simulink model "PV_Boost_Converter_PWM"  (R2020a)
settings: Solver=FixedStepAuto  StartTime=0.0  StopTime=0.5  FixedStep=1e-6  RelTol=1e-3
values from neighbouring files (symbols this model uses):
  Eg = 1.1    [data.m]
  Isc = 8.21    [data.m]
  k = 1.38*((10)^-23)    (= 1.38e-23)    [data.m]
  ki = 0.0032    [data.m]
  n = 1.3    [data.m]
  Ns = 54    [data.m]
  q = 1.6*((10)^-19)    (= 1.6e-19)    [data.m]
  Rs = 0.221    [data.m]
  Rsh = 415.405    [data.m]
  Tn = 298    [data.m]
  Voc = 32.9    [data.m]
libraries: powerlib x27, fuzblock x2, powerlib_meascontrol x2, re_lib x1
settings Model: Creator=Khojasteh Mirza  LastModifiedBy=Khojasteh Mirza

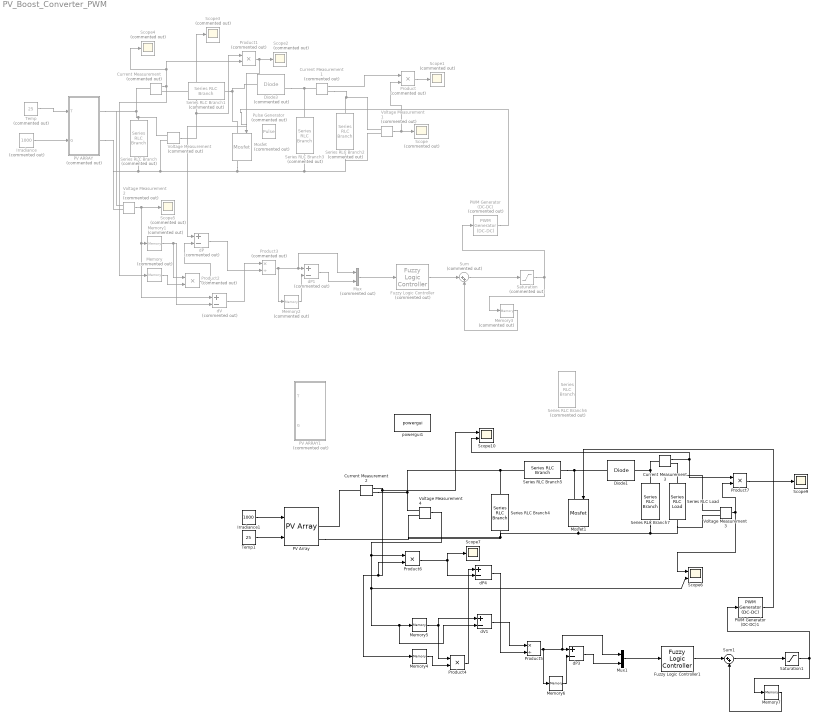
== system PV_Boost_Converter_PWM ==
  Current Measurement : powerlib/Measurements/Current Measurement  Commented=on  PhasorSimulation=off  OutputType=Complex  PSBequivalent=0
  Current Measurement1 : powerlib/Measurements/Current Measurement  Commented=on  PhasorSimulation=off  OutputType=Complex  PSBequivalent=0
  Current Measurement2 : powerlib/Measurements/Current Measurement  PhasorSimulation=off  OutputType=Complex  PSBequivalent=0
  Current Measurement3 : powerlib/Measurements/Current Measurement  PhasorSimulation=off  OutputType=Complex  PSBequivalent=0
  Diode1 : powerlib/Power Electronics/Diode  Ron=0.001  Lon=0  Vf=0.8  IC=0  UseSnubber=0  Rs=500  Cs=250e-9  Measurements=off
  Diode3 : powerlib/Power Electronics/Diode  Commented=on  Ron=0.001  Lon=0  Vf=0.8  IC=0  UseSnubber=0  Rs=500  Cs=250e-9  Measurements=on
  Fuzzy Logic Controller : fuzblock/Fuzzy Logic  Controller  Commented=on  FIS='fuzzy_mppt.fis'  OutputSampleNumber=101  DataType=double  FuzzifiedInputs=off  RuleFiringStrengths=off  RuleOutputs=off  AggregatedOutputs=off  SimulateUsing=Interpreted execution  OutOfRangeInputValueMessage=warning  NoRuleFiredMessage=warning  EmptyOutputFuzzySetMessage=warning
  Fuzzy Logic Controller1 : fuzblock/Fuzzy Logic  Controller  FIS='fuzzy_mppt.fis'  OutputSampleNumber=101  DataType=double  FuzzifiedInputs=off  RuleFiringStrengths=off  RuleOutputs=off  AggregatedOutputs=off  SimulateUsing=Interpreted execution  OutOfRangeInputValueMessage=warning  NoRuleFiredMessage=warning  EmptyOutputFuzzySetMessage=warning
  Irradiance : Constant  Commented=on  Value=1000
  Irradiance1 : Constant  Value=1000
  Memory{,1..3} (4 alike) : Memory  Commented=on
  Memory{4..7} (4 alike) : Memory
  Mosfet : powerlib/Power Electronics/Mosfet  Commented=on  Ron=0.1  Lon=0  Rd=0.01  Vfd=0  IC=0  Rs=1e5  Cs=inf  Measurements=on
  Mosfet1 : powerlib/Power Electronics/Mosfet  Ron=0.1  Lon=0  Rd=0.01  Vfd=0  IC=0  Rs=1e5  Cs=inf  Measurements=off
  Mux : Mux  Commented=on  Inputs=2
  Mux1 : Mux  Inputs=2
  PV ARRAY : Subsystem  Commented=on
  PV ARRAY1 : Subsystem  Commented=on
  PV Array : re_lib/Solar/PV Array  Npar=1  Nser=1  PlotType=array @ 25 deg.C & specified irradiances  S_vec=[1000]  Temp_C_vec=[800]  ModuleName=Kyocera Solar KC200GT  PlotWhenSelected=off  Pm=200.143  Ncell=54  Voc=32.9  Isc=8.21  Vm=26.3  Im=7.61  beta_Voc_pc=-0.35502  alpha_Isc_pc=0.06  beta_Voc=-0.1168  alpha_Isc=0.004926  IL=8.2288  I0=2.3246e-10  nI=0.97736  Rsh=150.6921  Rs=0.34483  RobustModel=off  RobustCellTemperature=25  BAL=on  Tc=1e-6  Tfilter=5e-5
  PWM Generator (DC-DC) : powerlib_meascontrol/Pulse & Signal Generators/PWM Generator (DC-DC)  Commented=on  Fsw=5000  Ts=0
  PWM Generator (DC-DC)1 : powerlib_meascontrol/Pulse & Signal Generators/PWM Generator (DC-DC)  Fsw=5000  Ts=0
  Product : Product  Commented=on
  Product1 : Product  Commented=on
  Product2 : Product  Commented=on
  Product3 : Product  Commented=on  Inputs=*/
  Product4 : Product
  Product5 : Product  Inputs=*/
  Product6 : Product
  Product7 : Product
  Pulse Generator : DiscretePulseGenerator  Commented=on  PulseType=Time based  Period=0.00004  PulseWidth=10
  Saturation : Saturate  Commented=on
  Saturation1 : Saturate
  Scope{,1..5} (6 alike) : Scope  Commented=on
  Scope10 : Scope  NumInputPorts=2
  Scope6 : Scope  NumInputPorts=2
  Scope7 : Scope
  Scope9 : Scope
  Series RLC Branch : powerlib/Elements/Series RLC Branch  Commented=on  LConnTagsString=__new0  RConnTagsString=__new0  BranchType=C  Resistance=1  Inductance=1e-3  SetiL0=off  InitialCurrent=0  Capacitance=1e-6  Setx0=off  InitialVoltage=0  Measurements=None
  Series RLC Branch1 : powerlib/Elements/Series RLC Branch  Commented=on  LConnTagsString=__new0  RConnTagsString=__new0  BranchType=L  Resistance=1  Inductance=650e-6  SetiL0=off  InitialCurrent=0  Capacitance=1e-6  Setx0=off  InitialVoltage=0  Measurements=None
  Series RLC Branch2 : powerlib/Elements/Series RLC Branch  Commented=on  LConnTagsString=__new0  RConnTagsString=__new0  BranchType=R  Resistance=10  Inductance=1e-3  SetiL0=off  InitialCurrent=0  Capacitance=1e-6  Setx0=off  InitialVoltage=0  Measurements=None
  Series RLC Branch3 : powerlib/Elements/Series RLC Branch  Commented=on  LConnTagsString=__new0  RConnTagsString=__new0  BranchType=C  Resistance=1  Inductance=1e-3  SetiL0=off  InitialCurrent=0  Capacitance=30e-6  Setx0=off  InitialVoltage=0  Measurements=None
  Series RLC Branch4 : powerlib/Elements/Series RLC Branch  LConnTagsString=__new0  RConnTagsString=__new0  BranchType=C  Resistance=1  Inductance=1e-3  SetiL0=off  InitialCurrent=0  Capacitance=4000e-6  Setx0=off  InitialVoltage=0  Measurements=None
  Series RLC Branch5 : powerlib/Elements/Series RLC Branch  LConnTagsString=__new0  RConnTagsString=__new0  BranchType=L  Resistance=1  Inductance=1e-4  SetiL0=off  InitialCurrent=0  Capacitance=1e-6  Setx0=off  InitialVoltage=0  Measurements=None
  Series RLC Branch6 : powerlib/Elements/Series RLC Branch  Commented=on  LConnTagsString=__new0  RConnTagsString=__new0  BranchType=R  Resistance=10  Inductance=1e-3  SetiL0=off  InitialCurrent=0  Capacitance=1e-6  Setx0=off  InitialVoltage=0  Measurements=None
  Series RLC Branch7 : powerlib/Elements/Series RLC Branch  LConnTagsString=__new0  RConnTagsString=__new0  BranchType=C  Resistance=1  Inductance=1e-3  SetiL0=off  InitialCurrent=0  Capacitance=50e-6  Setx0=off  InitialVoltage=0  Measurements=None
  Series RLC Load : powerlib/Elements/Series RLC Load  LConnTagsString=a  RConnTagsString=__new0  NominalVoltage=30  NominalFrequency=50  ActivePower=120  InductivePower=0  CapacitivePower=0  Setx0=off  InitialVoltage=0  SetiL0=off  InitialCurrent=0  Measurements=None  LoadType=constant Z
  Sum : Sum  Commented=on  Inputs=|++
  Sum1 : Sum  Inputs=|++
  Temp : Constant  Commented=on  Value=25
  Temp1 : Constant  Value=25
  Voltage Measurement : powerlib/Measurements/Voltage Measurement  Commented=on  PhasorSimulation=off  OutputType=Complex  PSBequivalent=0
  Voltage Measurement1 : powerlib/Measurements/Voltage Measurement  Commented=on  PhasorSimulation=off  OutputType=Complex  PSBequivalent=0
  Voltage Measurement2 : powerlib/Measurements/Voltage Measurement  Commented=on  PhasorSimulation=off  OutputType=Complex  PSBequivalent=0
  Voltage Measurement3 : powerlib/Measurements/Voltage Measurement  PhasorSimulation=off  OutputType=Complex  PSBequivalent=0
  Voltage Measurement4 : powerlib/Measurements/Voltage Measurement  PhasorSimulation=off  OutputType=Complex  PSBequivalent=0
  dP : Sum  Commented=on  Inputs=+-
  dP1 : Sum  Commented=on  Inputs=+-
  dP3 : Sum  Inputs=+-
  dP4 : Sum  Inputs=+-
  dV : Sum  Commented=on  Inputs=+-
  dV1 : Sum  Inputs=+-
  powergui1 : powerlib/powergui  Priority=1  SimulationMode=Discrete  SampleTime=5e-5  frequency=60  Iterations=50  frequencyindice=0  Pbase=100e6  ErrMax=1e-4  UnitsV=kV  UnitsW=MW  buscounter=0  FunctionMessages=off  echomessages=off  EnableUseOfTLC=off  CurrentSourceSwitches=off  DisableSnubberDevices=off  DisableRonSwitches=off  DisableVfSwitches=off  DisplayEquations=off  AutomaticDiscreteSolvers=off  SolverType=Tustin/Backward Euler (TBE)  Interpol=off  ExternalGateDelay=off  methode=off  Ts=100  x0status=blocks  SPID=on  SwTol=0  HookPort=off  NonlinearTolerance=1e-4  nMaxIteration=100  ContinueOnMaxIteration=off  RestoreLinks=warning  ResistiveCurrentMeasurement=off  Frange=[0:2:500]  Ylog=off  Xlog=on  ShowGrid=off  save=off  variable=ZData  structure=0  ZoomFFT=off  StartTime=0.0  cycles=1  DisplayStyle=1  fundamental=60  FreqAxis=off  MaxFrequency=1000  frequencyindicesteady=1  RmsSteady=1  display=off
  wires:
  Temp/1 -> PV ARRAY/1(T)
  Irradiance/1 -> PV ARRAY/2(G)
  Voltage Measurement1/1 -> Product/2, Scope/1
  Current Measurement1/1 -> Product/1
  Product/1 -> Scope1/1
  Product1/1 -> dP/1, Scope2/1
  Voltage Measurement/1 -> Scope3/1, Product1/1
  Current Measurement/1 -> Scope4/1, Product1/2, Memory/1
  Voltage Measurement2/1 -> dV/1, Memory1/1, Scope5/1
  Memory1/1 -> dV/2, Product2/1
  Memory/1 -> Product2/2
  Product2/1 -> dP/2
  dV/1 -> Product3/1
  dP/1 -> Product3/2
  Product3/1 -> Memory2/1, Mux/1, dP1/1
  Memory2/1 -> dP1/2
  dP1/1 -> Mux/2
  Mux/1 -> Fuzzy Logic Controller/1
  Fuzzy Logic Controller/1 -> Sum/1
  Sum/1 -> Saturation/1
  Saturation/1 -> PWM Generator (DC-DC)/1, Memory3/1
  Memory3/1 -> Sum/2
  PWM Generator (DC-DC)/1 -> Mosfet/1
  Memory4/1 -> Product4/2
  Memory7/1 -> Sum1/2
  Sum1/1 -> Saturation1/1
  Product4/1 -> dP4/1
  dP3/1 -> Mux1/2
  Saturation1/1 -> PWM Generator (DC-DC)1/1, Memory7/1
  dV1/1 -> Product5/1
  Memory6/1 -> dP3/2
  Mux1/1 -> Fuzzy Logic Controller1/1
  Fuzzy Logic Controller1/1 -> Sum1/1
  Memory5/1 -> dV1/1, Product4/1
  Product5/1 -> Memory6/1, Mux1/1, dP3/1
  Current Measurement2/1 -> Scope10/1, Memory4/1, Product6/2
  Product6/1 -> Scope7/1, dP4/2
  dP4/1 -> Product5/2
  PWM Generator (DC-DC)1/1 -> Mosfet1/1
  Voltage Measurement3/1 -> Product7/2, Scope6/1
  Irradiance1/1 -> PV Array/1
  Temp1/1 -> PV Array/2
  Current Measurement3/1 -> Product7/1, Scope10/2
  Product7/1 -> Scope9/1
  Voltage Measurement4/1 -> Scope6/2, dV1/2, Memory5/1, Product6/1
  connections:
  Current Measurement/LConn1 -- Voltage Measurement2/LConn1 -- PV ARRAY/RConn1 -- Series RLC Branch/LConn1 -- Voltage Measurement/LConn1
  Series RLC Branch1/LConn1 -- Current Measurement/RConn1
  Series RLC Branch2/LConn1 -- Current Measurement1/RConn1 -- Voltage Measurement1/LConn1
  Series RLC Branch3/LConn1 -- Diode3/RConn1 -- Current Measurement1/LConn1
  Series RLC Branch3/RConn1 -- Mosfet/RConn1 -- Series RLC Branch/RConn1 -- PV ARRAY/RConn2 -- Voltage Measurement2/LConn2 -- Voltage Measurement/LConn2 -- Voltage Measurement1/LConn2 -- Series RLC Branch2/RConn1
  Series RLC Branch1/RConn1 -- Diode3/LConn1 -- Mosfet/LConn1
  Series RLC Branch5/RConn1 -- Diode1/LConn1 -- Mosfet1/LConn1
  Voltage Measurement3/LConn1 -- Current Measurement3/RConn1 -- Series RLC Load/LConn1
  Current Measurement2/RConn1 -- Series RLC Branch4/LConn1 -- Series RLC Branch5/LConn1 -- Voltage Measurement4/LConn1
  Series RLC Branch4/RConn1 -- Voltage Measurement4/LConn2 -- PV Array/RConn2 -- Voltage Measurement3/LConn2 -- Series RLC Load/RConn1 -- Series RLC Branch7/RConn1 -- Mosfet1/RConn1
  Current Measurement2/LConn1 -- PV Array/RConn1
  Series RLC Branch7/LConn1 -- Current Measurement3/LConn1 -- Diode1/RConn1

== system PV_Boost_Converter_PWM/PV ARRAY ==
  T : Inport
  G : Inport  Port=2
  Controlled Current Source : powerlib/Electrical Sources/Controlled Current Source  Initialize=on  Source_Type=AC  Amplitude=0  Phase=0  Frequency=0  Measurements=None
  PV Module : Subsystem
  Voltage Measurement : powerlib/Measurements/Voltage Measurement  PhasorSimulation=off  OutputType=Complex  PSBequivalent=0
  + : PMIOPort  Side=Right
  - : PMIOPort  Port=2  Side=Right
  wires:
  G/1 -> PV Module/2(G)
  Voltage Measurement/1 -> PV Module/3(Varray)
  T/1 -> PV Module/1(T)
  PV Module/1(I) -> Controlled Current Source/1
  connections:
  Controlled Current Source/LConn1 -- -/RConn1 -- Voltage Measurement/LConn2
  Controlled Current Source/RConn1 -- +/RConn1 -- Voltage Measurement/LConn1

== system PV_Boost_Converter_PWM/PV ARRAY1 ==
  T : Inport
  G : Inport  Port=2
  Controlled Current Source : powerlib/Electrical Sources/Controlled Current Source  Initialize=on  Source_Type=AC  Amplitude=0  Phase=0  Frequency=0  Measurements=None
  PV Module : Subsystem
  Voltage Measurement : powerlib/Measurements/Voltage Measurement  PhasorSimulation=off  OutputType=Complex  PSBequivalent=0
  + : PMIOPort  Side=Right
  - : PMIOPort  Port=2  Side=Right
  wires:
  G/1 -> PV Module/2(G)
  Voltage Measurement/1 -> PV Module/3(Varray)
  T/1 -> PV Module/1(T)
  PV Module/1(I) -> Controlled Current Source/1
  connections:
  Controlled Current Source/LConn1 -- -/RConn1 -- Voltage Measurement/LConn2
  Controlled Current Source/RConn1 -- +/RConn1 -- Voltage Measurement/LConn1

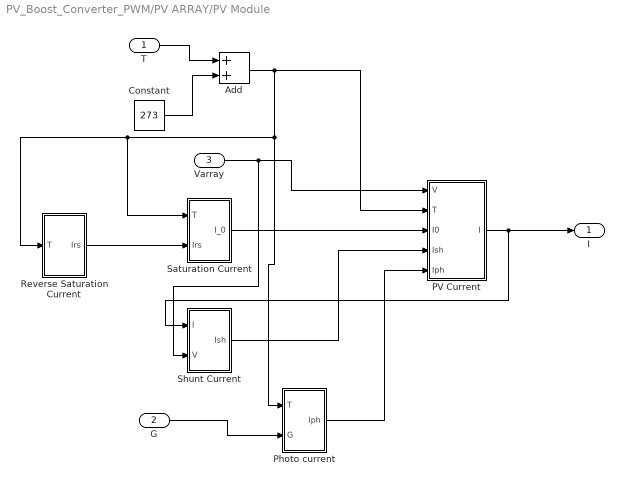
== system PV_Boost_Converter_PWM/PV ARRAY/PV Module ==
  T : Inport
  G : Inport  Port=2
  Varray : Inport  Port=3
  Add : Sum
  Constant : Constant  Value=273
  PV Current : Subsystem
  Photo current : Subsystem
  Reverse Saturation Current : Subsystem
  Saturation Current : Subsystem
  Shunt Current : Subsystem
  I : Outport
  wires:
  Shunt Current/1(Ish) -> PV Current/4(Ish)
  Varray/1 -> Shunt Current/2(V), PV Current/1(V)
  Reverse Saturation Current/1(Irs) -> Saturation Current/2(Irs)
  Saturation Current/1(I_0) -> PV Current/3(I0)
  Constant/1 -> Add/2
  G/1 -> Photo current/2(G)
  T/1 -> Add/1
  PV Current/1(I) -> I/1, Shunt Current/1(I)
  Photo current/1(Iph) -> PV Current/5(Iph)
  Add/1 -> Saturation Current/1(T), Reverse Saturation Current/1(T), Photo current/1(T), PV Current/2(T)

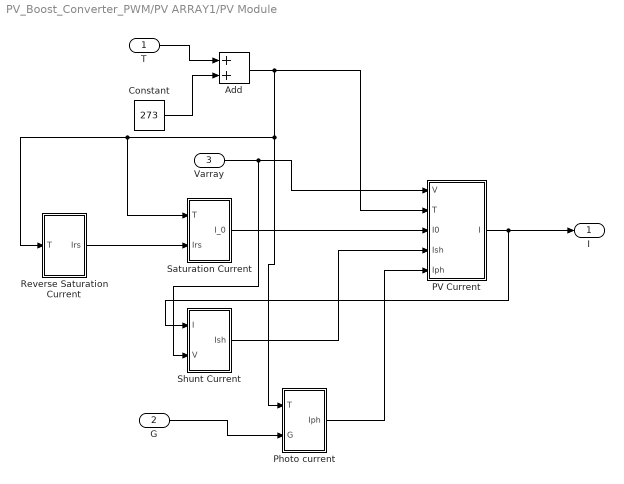
== system PV_Boost_Converter_PWM/PV ARRAY1/PV Module ==
  T : Inport
  G : Inport  Port=2
  Varray : Inport  Port=3
  Add : Sum
  Constant : Constant  Value=273
  PV Current : Subsystem
  Photo current : Subsystem
  Reverse Saturation Current : Subsystem
  Saturation Current : Subsystem
  Shunt Current : Subsystem
  I : Outport
  wires:
  Shunt Current/1(Ish) -> PV Current/4(Ish)
  Varray/1 -> Shunt Current/2(V), PV Current/1(V)
  Reverse Saturation Current/1(Irs) -> Saturation Current/2(Irs)
  Saturation Current/1(I_0) -> PV Current/3(I0)
  Constant/1 -> Add/2
  G/1 -> Photo current/2(G)
  T/1 -> Add/1
  PV Current/1(I) -> I/1, Shunt Current/1(I)
  Photo current/1(Iph) -> PV Current/5(Iph)
  Add/1 -> Saturation Current/1(T), Reverse Saturation Current/1(T), Photo current/1(T), PV Current/2(T)

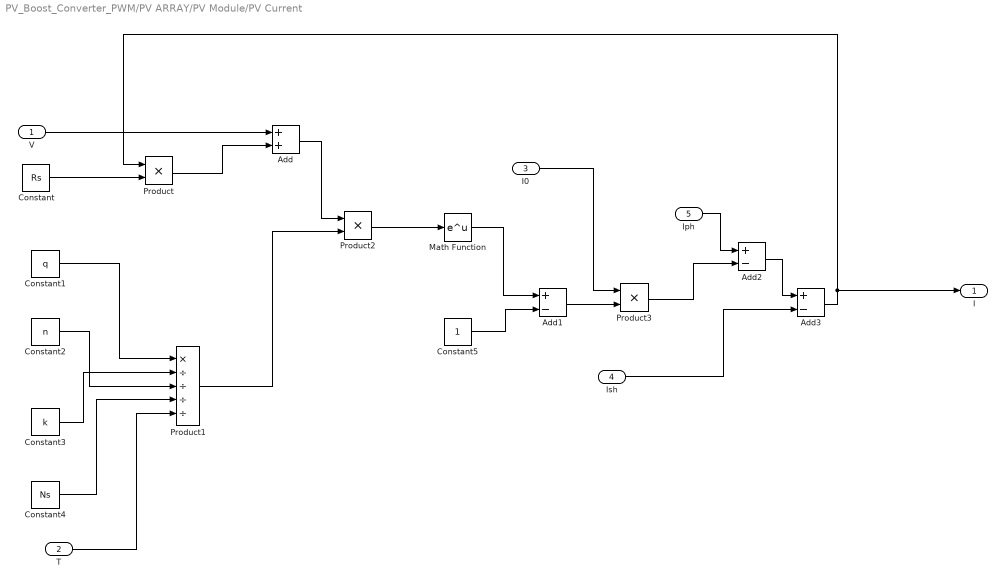
== system PV_Boost_Converter_PWM/PV ARRAY/PV Module/PV Current ==
  V : Inport
  T : Inport  Port=2
  I0 : Inport  Port=3
  Ish : Inport  Port=4
  Iph : Inport  Port=5
  Add : Sum
  Add1 : Sum  Inputs=+-
  Add2 : Sum  Inputs=+-
  Add3 : Sum  Inputs=+-
  Constant : Constant  Value=Rs
  Constant1 : Constant  Value=q
  Constant2 : Constant  Value=n
  Constant3 : Constant  Value=k
  Constant4 : Constant  Value=Ns
  Constant5 : Constant
  Math Function : Math  SaturateOnIntegerOverflow=on
  Product : Product
  Product1 : Product  Inputs=*////
  Product2 : Product
  Product3 : Product
  I : Outport
  wires:
  Constant3/1 -> Product1/2
  Constant/1 -> Product/2
  Math Function/1 -> Add1/1
  Iph/1 -> Add2/1
  Product2/1 -> Math Function/1
  I0/1 -> Product3/1
  Ish/1 -> Add3/2
  Product/1 -> Add/2
  Constant4/1 -> Product1/4
  Add/1 -> Product2/1
  Add3/1 -> I/1, Product/1
  Add1/1 -> Product3/2
  Constant2/1 -> Product1/3
  Add2/1 -> Add3/1
  T/1 -> Product1/5
  Product3/1 -> Add2/2
  V/1 -> Add/1
  Constant1/1 -> Product1/1
  Constant5/1 -> Add1/2
  Product1/1 -> Product2/2

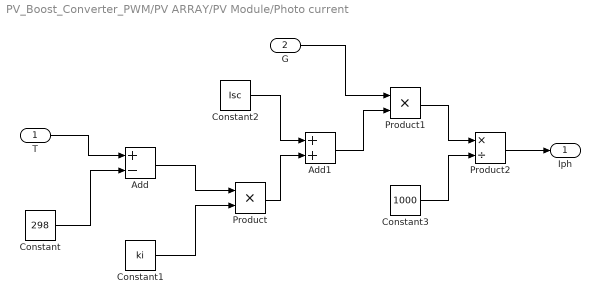
== system PV_Boost_Converter_PWM/PV ARRAY/PV Module/Photo current ==
  T : Inport
  G : Inport  Port=2
  Add : Sum  Inputs=+-
  Add1 : Sum
  Constant : Constant  Value=298
  Constant1 : Constant  Value=ki
  Constant2 : Constant  Value=Isc
  Constant3 : Constant  Value=1000
  Product : Product
  Product1 : Product
  Product2 : Product  Inputs=*/
  Iph : Outport
  wires:
  Add/1 -> Product/1
  T/1 -> Add/1
  Constant2/1 -> Add1/1
  Constant/1 -> Add/2
  Product/1 -> Add1/2
  Constant1/1 -> Product/2
  G/1 -> Product1/1
  Constant3/1 -> Product2/2
  Add1/1 -> Product1/2
  Product1/1 -> Product2/1
  Product2/1 -> Iph/1

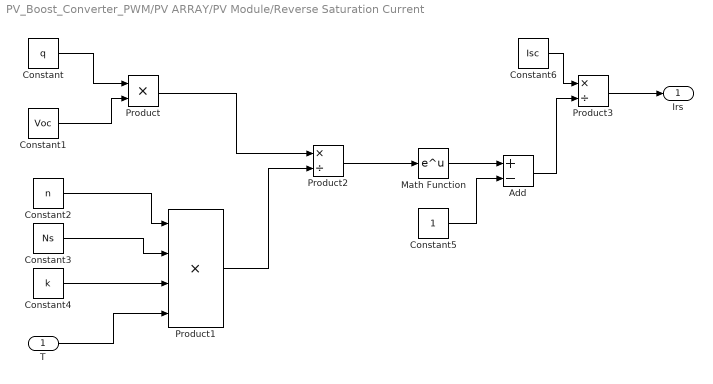
== system PV_Boost_Converter_PWM/PV ARRAY/PV Module/Reverse Saturation Current ==
  T : Inport
  Add : Sum  Inputs=+-
  Constant : Constant  Value=q
  Constant1 : Constant  Value=Voc
  Constant2 : Constant  Value=n
  Constant3 : Constant  Value=Ns
  Constant4 : Constant  Value=k
  Constant5 : Constant
  Constant6 : Constant  Value=Isc
  Math Function : Math  SaturateOnIntegerOverflow=on
  Product : Product
  Product1 : Product  Inputs=4
  Product2 : Product  Inputs=*/
  Product3 : Product  Inputs=*/
  Irs : Outport
  wires:
  Constant6/1 -> Product3/1
  Add/1 -> Product3/2
  Constant5/1 -> Add/2
  Constant3/1 -> Product1/2
  Product3/1 -> Irs/1
  Product1/1 -> Product2/2
  Math Function/1 -> Add/1
  Product/1 -> Product2/1
  Constant2/1 -> Product1/1
  Product2/1 -> Math Function/1
  Constant/1 -> Product/1
  Constant1/1 -> Product/2
  T/1 -> Product1/4
  Constant4/1 -> Product1/3

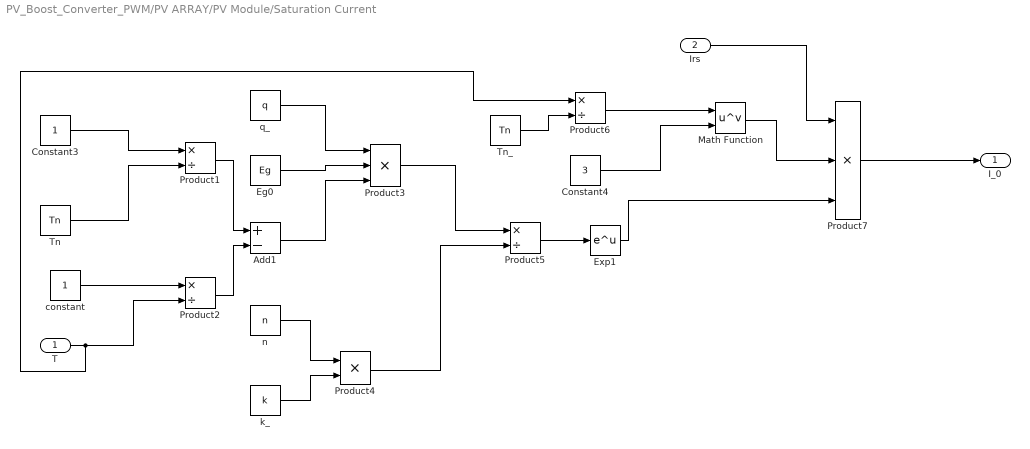
== system PV_Boost_Converter_PWM/PV ARRAY/PV Module/Saturation Current ==
  T : Inport
  Irs : Inport  Port=2
  Add1 : Sum  Inputs=+-
  Constant3 : Constant
  Constant4 : Constant  Value=3
  Eg0 : Constant  Value=Eg
  Exp1 : Math  SaturateOnIntegerOverflow=on
  Math Function : Math  Operator=pow  SaturateOnIntegerOverflow=on
  Product{1..2,5..6} (4 alike) : Product  Inputs=*/
  Product3 : Product  Inputs=***
  Product4 : Product  Inputs=**
  Product7 : Product  Inputs=3
  Tn : Constant  Value=Tn
  Tn_ : Constant  Value=Tn
  constant : Constant
  k_ : Constant  Value=k
  n : Constant  Value=n
  q_ : Constant  Value=q
  I_0 : Outport
  wires:
  T/1 -> Product2/2, Product6/1
  Product1/1 -> Add1/1
  constant/1 -> Product2/1
  Irs/1 -> Product7/1
  Tn_/1 -> Product6/2
  Product5/1 -> Exp1/1
  Product3/1 -> Product5/1
  q_/1 -> Product3/1
  Exp1/1 -> Product7/3
  Product2/1 -> Add1/2
  Product4/1 -> Product5/2
  Constant4/1 -> Math Function/2
  Math Function/1 -> Product7/2
  Tn/1 -> Product1/2
  Product6/1 -> Math Function/1
  k_/1 -> Product4/2
  Constant3/1 -> Product1/1
  Eg0/1 -> Product3/2
  n/1 -> Product4/1
  Add1/1 -> Product3/3
  Product7/1 -> I_0/1

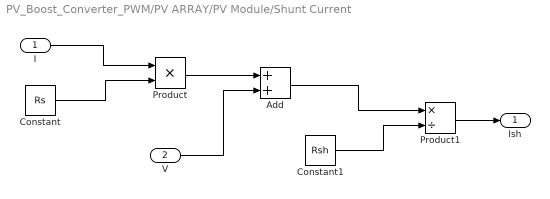
== system PV_Boost_Converter_PWM/PV ARRAY/PV Module/Shunt Current ==
  I : Inport
  V : Inport  Port=2
  Add : Sum
  Constant : Constant  Value=Rs
  Constant1 : Constant  Value=Rsh
  Product : Product
  Product1 : Product  Inputs=*/
  Ish : Outport
  wires:
  Product1/1 -> Ish/1
  Constant/1 -> Product/2
  Constant1/1 -> Product1/2
  V/1 -> Add/2
  Product/1 -> Add/1
  Add/1 -> Product1/1
  I/1 -> Product/1

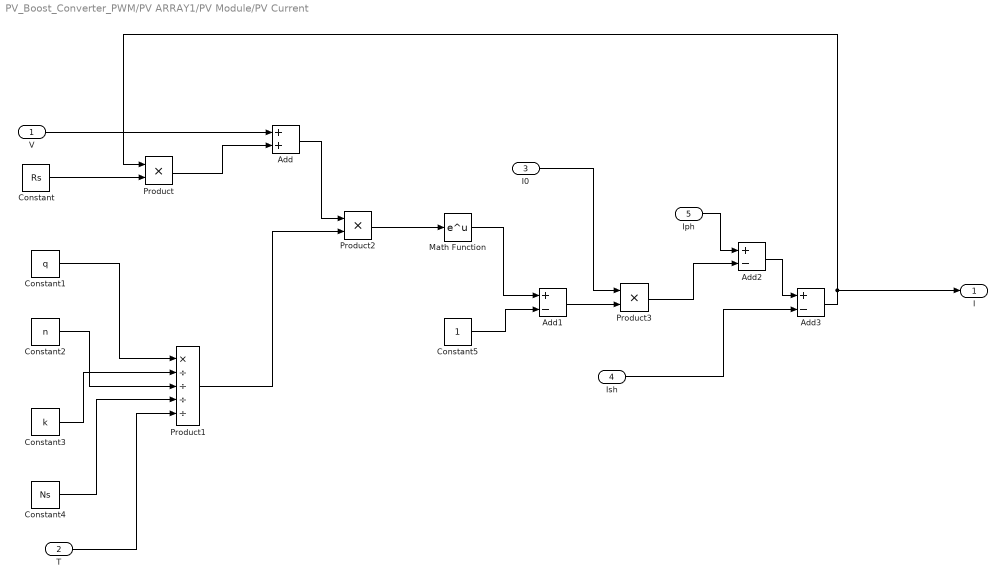
== system PV_Boost_Converter_PWM/PV ARRAY1/PV Module/PV Current ==
  V : Inport
  T : Inport  Port=2
  I0 : Inport  Port=3
  Ish : Inport  Port=4
  Iph : Inport  Port=5
  Add : Sum
  Add1 : Sum  Inputs=+-
  Add2 : Sum  Inputs=+-
  Add3 : Sum  Inputs=+-
  Constant : Constant  Value=Rs
  Constant1 : Constant  Value=q
  Constant2 : Constant  Value=n
  Constant3 : Constant  Value=k
  Constant4 : Constant  Value=Ns
  Constant5 : Constant
  Math Function : Math  SaturateOnIntegerOverflow=on
  Product : Product
  Product1 : Product  Inputs=*////
  Product2 : Product
  Product3 : Product
  I : Outport
  wires:
  Constant3/1 -> Product1/2
  Constant/1 -> Product/2
  Math Function/1 -> Add1/1
  Iph/1 -> Add2/1
  Product2/1 -> Math Function/1
  I0/1 -> Product3/1
  Ish/1 -> Add3/2
  Product/1 -> Add/2
  Constant4/1 -> Product1/4
  Add/1 -> Product2/1
  Add3/1 -> I/1, Product/1
  Add1/1 -> Product3/2
  Constant2/1 -> Product1/3
  Add2/1 -> Add3/1
  T/1 -> Product1/5
  Product3/1 -> Add2/2
  V/1 -> Add/1
  Constant1/1 -> Product1/1
  Constant5/1 -> Add1/2
  Product1/1 -> Product2/2

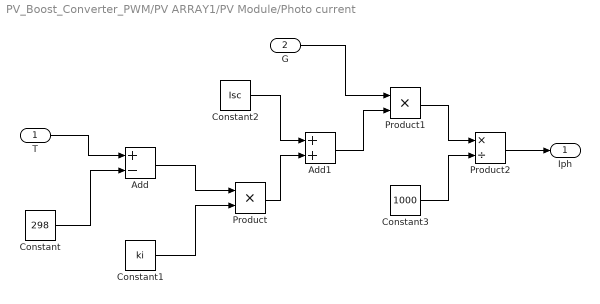
== system PV_Boost_Converter_PWM/PV ARRAY1/PV Module/Photo current ==
  T : Inport
  G : Inport  Port=2
  Add : Sum  Inputs=+-
  Add1 : Sum
  Constant : Constant  Value=298
  Constant1 : Constant  Value=ki
  Constant2 : Constant  Value=Isc
  Constant3 : Constant  Value=1000
  Product : Product
  Product1 : Product
  Product2 : Product  Inputs=*/
  Iph : Outport
  wires:
  Add/1 -> Product/1
  T/1 -> Add/1
  Constant2/1 -> Add1/1
  Constant/1 -> Add/2
  Product/1 -> Add1/2
  Constant1/1 -> Product/2
  G/1 -> Product1/1
  Constant3/1 -> Product2/2
  Add1/1 -> Product1/2
  Product1/1 -> Product2/1
  Product2/1 -> Iph/1

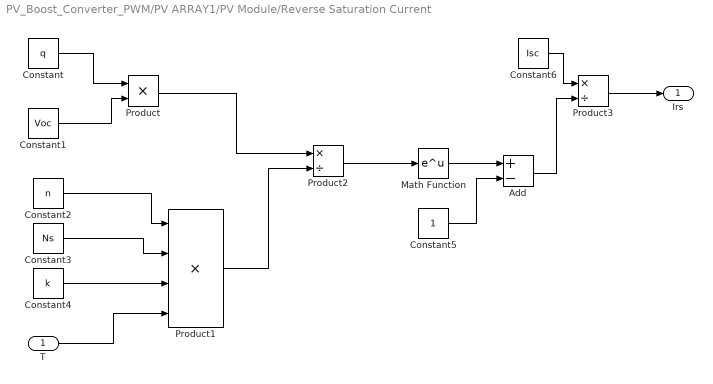
== system PV_Boost_Converter_PWM/PV ARRAY1/PV Module/Reverse Saturation Current ==
  T : Inport
  Add : Sum  Inputs=+-
  Constant : Constant  Value=q
  Constant1 : Constant  Value=Voc
  Constant2 : Constant  Value=n
  Constant3 : Constant  Value=Ns
  Constant4 : Constant  Value=k
  Constant5 : Constant
  Constant6 : Constant  Value=Isc
  Math Function : Math  SaturateOnIntegerOverflow=on
  Product : Product
  Product1 : Product  Inputs=4
  Product2 : Product  Inputs=*/
  Product3 : Product  Inputs=*/
  Irs : Outport
  wires:
  Constant6/1 -> Product3/1
  Add/1 -> Product3/2
  Constant5/1 -> Add/2
  Constant3/1 -> Product1/2
  Product3/1 -> Irs/1
  Product1/1 -> Product2/2
  Math Function/1 -> Add/1
  Product/1 -> Product2/1
  Constant2/1 -> Product1/1
  Product2/1 -> Math Function/1
  Constant/1 -> Product/1
  Constant1/1 -> Product/2
  T/1 -> Product1/4
  Constant4/1 -> Product1/3

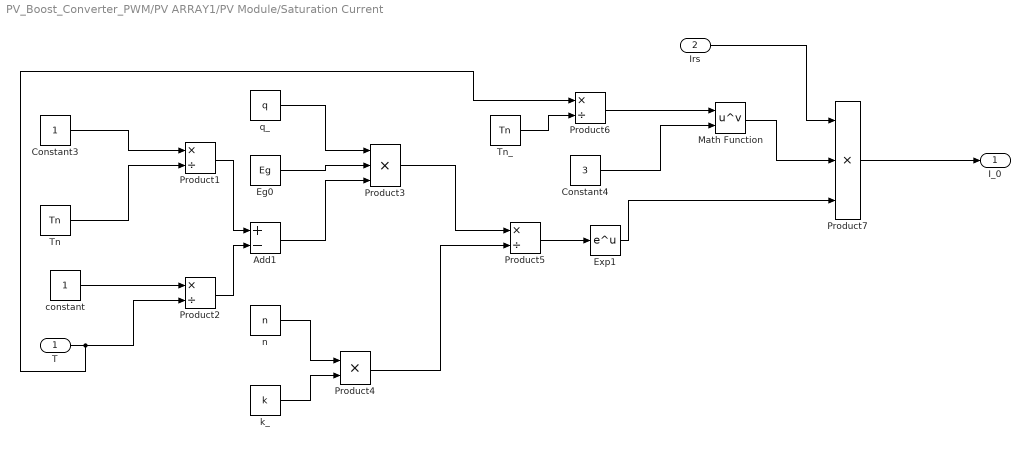
== system PV_Boost_Converter_PWM/PV ARRAY1/PV Module/Saturation Current ==
  T : Inport
  Irs : Inport  Port=2
  Add1 : Sum  Inputs=+-
  Constant3 : Constant
  Constant4 : Constant  Value=3
  Eg0 : Constant  Value=Eg
  Exp1 : Math  SaturateOnIntegerOverflow=on
  Math Function : Math  Operator=pow  SaturateOnIntegerOverflow=on
  Product{1..2,5..6} (4 alike) : Product  Inputs=*/
  Product3 : Product  Inputs=***
  Product4 : Product  Inputs=**
  Product7 : Product  Inputs=3
  Tn : Constant  Value=Tn
  Tn_ : Constant  Value=Tn
  constant : Constant
  k_ : Constant  Value=k
  n : Constant  Value=n
  q_ : Constant  Value=q
  I_0 : Outport
  wires:
  T/1 -> Product2/2, Product6/1
  Product1/1 -> Add1/1
  constant/1 -> Product2/1
  Irs/1 -> Product7/1
  Tn_/1 -> Product6/2
  Product5/1 -> Exp1/1
  Product3/1 -> Product5/1
  q_/1 -> Product3/1
  Exp1/1 -> Product7/3
  Product2/1 -> Add1/2
  Product4/1 -> Product5/2
  Constant4/1 -> Math Function/2
  Math Function/1 -> Product7/2
  Tn/1 -> Product1/2
  Product6/1 -> Math Function/1
  k_/1 -> Product4/2
  Constant3/1 -> Product1/1
  Eg0/1 -> Product3/2
  n/1 -> Product4/1
  Add1/1 -> Product3/3
  Product7/1 -> I_0/1

== system PV_Boost_Converter_PWM/PV ARRAY1/PV Module/Shunt Current ==
  I : Inport
  V : Inport  Port=2
  Add : Sum
  Constant : Constant  Value=Rs
  Constant1 : Constant  Value=Rsh
  Product : Product
  Product1 : Product  Inputs=*/
  Ish : Outport
  wires:
  Product1/1 -> Ish/1
  Constant/1 -> Product/2
  Constant1/1 -> Product1/2
  V/1 -> Add/2
  Product/1 -> Add/1
  Add/1 -> Product1/1
  I/1 -> Product/1
